simulink library "dspsolvers"  (Simulink 8.0)
settings: Solver=ode45  SolverMode=SingleTasking  StartTime=0.0  StopTime=10.0  RelTol=1e-3
values from neighbouring files (symbols this model uses):
  D = D + B    [rebuffer_delay.m]
libraries: dspsigattribs x12, dspsolvers x6, dspfactors x3, dspmtrx3 x3, dspinverses x1
settings Model: Creator=dlinebar  LastModifiedBy=amoyer  CovMetricSettings=d  ExtModeAutoUpdateStatusClock=off

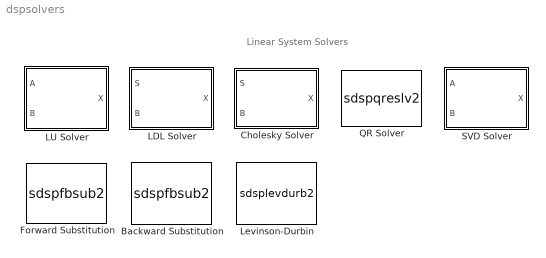
== system dspsolvers ==
  note: Linear System Solvers
  Backward Substitution : S-Function  DialogController=SPCUnifiedFixptDlgDDG.FBSubst  DialogControllerArgs=DataTag0  FunctionName=sdspfbsub2  Parameters=Unit,RealDiag,1,outputMin,outputMax,dtInfo.prodOutputMode,dtInfo.prodOutputWordLength,dtInfo.prodOutputFracLength,dtInfo.accumMode,dtInfo.accumWordLength,dtInfo.accumFracLength,dtInfo.outputMode,dtInfo.outputWordLength,dtInfo.outputFracLength,dtInfo.roundingMode,dtInfo.overflowMode  EnableBusSupport=off  mask(Backward Substitution){Unit=off, RealDiag=off, outputMode=Same as first input, outputWordLength=16, outputFracLength=15, outputDataTypeStr=Inherit: Same as first input, outputLastDataTypeStr=Inherit: Same as first input, outputMin=[], outputMax=[], accumMode=Inherit via internal rule, accumWordLength=32, accumFracLength=30, accumDataTypeStr=Inherit: Inherit via internal rule, accumLastDataTypeStr=Inherit: Inherit via internal rule, prodOutputMode=Inherit via internal rule, prodOutputWordLength=32, prodOutputFracLength=30, prodOutputDataTypeStr=Inherit: Inherit via internal rule, prodOutputLastDataTypeStr=Inherit: Inherit via internal rule, roundingMode=Floor, overflowMode=off, LockScale=off}
      mask prompts: Unit "Input U is unit-upper triangular"; RealDiag "Diagonal of complex input U is real"; outputMode "Fixed-point output attributes:"; outputWordLength "Output word length:"; outputFracLength "Output fraction length:"; outputDataTypeStr "Output data type:"; outputLastDataTypeStr "Last output data type:"; outputMin "Output minimum:"; outputMax "Output maximum:"; accumMode "Fixed-point accumulator attributes:"; accumWordLength "Accumulator word length:"; accumFracLength "Accumulator fraction length:"; accumDataTypeStr "Accumulator data type:"; accumLastDataTypeStr "Last accumulator data type:"; prodOutputMode "Fixed-point product output attributes:"; prodOutputWordLength "Product output word length:"; prodOutputFracLength "Product output fraction length:"; prodOutputDataTypeStr "Product output data type:"; prodOutputLastDataTypeStr "Last product output data type:"; roundingMode "Round integer calculations toward:"; overflowMode "Saturate on integer overflow:"; LockScale "Lock scaling"
      mask help: dsp:dspsolvers:BackwardSubstitution_MD
      mask init:
      | blkh   = gcbh;
      | dtRows = dspblkGetFBSubstDTRowInfo();
      | dtInfo = dspGetUDTFixptDataTypeInfo(blkh, dtRows, true);
      mask Help: eval('blocksethelp');
      mask TypeOptions outputMode: Same as first input | Binary point scaling | Slope and bias scaling
      mask TypeOptions accumMode: Inherit via internal rule | Same as product output | Same as first input | Binary point scaling | Slope and bias scaling
      mask TypeOptions prodOutputMode: Inherit via internal rule | Same as first input | Binary point scaling | Slope and bias scaling
      mask TypeOptions roundingMode: Ceiling | Convergent | Floor | Nearest | Round | Simplest | Zero
      mask Display:
      | x=[ 0.45 0.45 0.18 0.45 NaN 0.495 0.585 0.585 0.495 0.495 NaN 0.63 0.675 NaN 0.63 0.675 NaN 0.72 0.81 0.81 0.72 0.72 ];
      | y=[ 0.1 0.7 0.7 0.1 NaN 0.1 0.1 0.7 0.7 0.1 NaN 0.35 0.35 NaN 0.45 0.45 NaN 0.1 0.1 0.7 0.7 0.1 ];
      | plot(x,y); text(.4,0.9,'U X = B');
      | port_label('input',1,'U');
      | port_label('input',2,'B');
      | port_label('output',1,'X');
  Cholesky Solver : Subsystem  mask(Cholesky Solver){errmode=Warning}
      mask prompts: errmode "dsp:dspsolvers:NonpositiveDefiniteInput_MP"
      mask help: dsp:dspsolvers:CholeskySolver_MD
      mask init:
      | x=[ 0.135 0.475 .475 0.135 0.135 NaN .135 .475 NaN 0.55 0.64 0.64 0.55  0.55 NaN 0.685 0.73 NaN 0.685 0.73 NaN 0.775 0.865 0.865 0.775 0.775 ];
      | y=[ 0.2 0.2 0.7 0.7 .2 NaN .7 .2 NaN 0.2 0.2 0.7 0.7 0.2 NaN 0.4 0.4 NaN 0.45 0.45 NaN 0.2 0.2 0.7 0.7 0.2 ];
      | set_param([gcb '/Cholesky Factorization'],'MaskTunableValues', {'off'});
      | set_param([gcb '/Cholesky Factorization'],'errmode',get_param(gcb,'errmode'));
      mask Help: eval('blocksethelp');
      mask TypeOptions errmode: dsp:dspsolvers:Ignore_CB | dsp:dspsolvers:Warning_CB | dsp:dspsolvers:Error_CB
      mask Display:
      | plot(x,y+0.05);
      | text(0.17,0.9,'SX=B (Chol)');
      | text(0.12,0.15,'[m x m]');
  Forward Substitution : S-Function  DialogController=SPCUnifiedFixptDlgDDG.FBSubst  DialogControllerArgs=DataTag1  FunctionName=sdspfbsub2  Parameters=Unit,RealDiag,0,outputMin,outputMax,dtInfo.prodOutputMode,dtInfo.prodOutputWordLength,dtInfo.prodOutputFracLength,dtInfo.accumMode,dtInfo.accumWordLength,dtInfo.accumFracLength,dtInfo.outputMode,dtInfo.outputWordLength,dtInfo.outputFracLength,dtInfo.roundingMode,dtInfo.overflowMode  EnableBusSupport=off  mask(Forward Substitution){Unit=off, RealDiag=off, outputMode=Same as first input, outputWordLength=16, outputFracLength=15, outputDataTypeStr=Inherit: Same as first input, outputLastDataTypeStr=Inherit: Same as first input, outputMin=[], outputMax=[], accumMode=Inherit via internal rule, accumWordLength=32, accumFracLength=30, accumDataTypeStr=Inherit: Inherit via internal rule, accumLastDataTypeStr=Inherit: Inherit via internal rule, prodOutputMode=Inherit via internal rule, prodOutputWordLength=32, prodOutputFracLength=30, prodOutputDataTypeStr=Inherit: Inherit via internal rule, prodOutputLastDataTypeStr=Inherit: Inherit via internal rule, roundingMode=Floor, overflowMode=off, LockScale=off}
      mask prompts: Unit "Input L is unit-lower triangular"; RealDiag "Diagonal of complex input L is real"; outputMode "Fixed-point output attributes:"; outputWordLength "Output word length:"; outputFracLength "Output fraction length:"; outputDataTypeStr "Output data type:"; outputLastDataTypeStr "Last output data type:"; outputMin "Output minimum:"; outputMax "Output maximum:"; accumMode "Fixed-point accumulator attributes:"; accumWordLength "Accumulator word length:"; accumFracLength "Accumulator fraction length:"; accumDataTypeStr "Accumulator data type:"; accumLastDataTypeStr "Last accumulator data type:"; prodOutputMode "Fixed-point product output attributes:"; prodOutputWordLength "Product output word length:"; prodOutputFracLength "Product output fraction length:"; prodOutputDataTypeStr "Product output data type:"; prodOutputLastDataTypeStr "Last product output data type:"; roundingMode "Round integer calculations toward:"; overflowMode "Saturate on integer overflow"; LockScale "Lock scaling"
      mask help: dsp:dspsolvers:ForwardSubstitution_MD
      mask init:
      | blkh   = gcbh;
      | dtRows = dspblkGetFBSubstDTRowInfo();
      | dtInfo = dspGetUDTFixptDataTypeInfo(blkh, dtRows, true);
      mask Help: eval('blocksethelp');
      mask TypeOptions outputMode: Same as first input | Binary point scaling | Slope and bias scaling
      mask TypeOptions accumMode: Inherit via internal rule | Same as product output | Same as first input | Binary point scaling | Slope and bias scaling
      mask TypeOptions prodOutputMode: Inherit via internal rule | Same as first input | Binary point scaling | Slope and bias scaling
      mask TypeOptions roundingMode: Ceiling | Convergent | Floor | Nearest | Round | Simplest | Zero
      mask Display:
      | x=[ 0.18 0.45 0.18 0.18 NaN 0.495 0.585 0.585 0.495 0.495 NaN 0.63 0.675 NaN 0.63 0.675 NaN 0.72 0.81 0.81 0.72 0.72 ];
      | y=[ 0.1 0.1 0.7 0.1 NaN 0.1 0.1 0.7 0.7 0.1 NaN 0.35 0.35 NaN 0.45 0.45 NaN 0.1 0.1 0.7 0.7 0.1 ];
      | plot(x,y); text(.4,0.9,'L X = B');
      | port_label('input',1,'L');
      | port_label('input',2,'B');
      | port_label('output',1,'X');
  LDL Solver : Subsystem  mask(LDL Solver){errmode=Warning}
      mask prompts: errmode "dsp:dspsolvers:NonpositiveDefiniteInput_MP"
      mask help: dsp:dspsolvers:LDLSolver_MD
      mask init:
      | Bcols=1;
      | x=[ 0.135 0.475 .475 0.135 0.135 NaN .135 .475 NaN 0.55 0.64 0.64 0.55 0.55 NaN 0.685 0.73 NaN 0.685 0.73 NaN 0.775 0.865 0.865 0.775 0.775 ];
      | y=[ 0.2 0.2 0.7 0.7 0.2 NaN .7 .2 NaN 0.2 0.2 0.7 0.7 0.2 NaN 0.4 0.4 NaN 0.45 0.45 NaN 0.2 0.2 0.7 0.7 0.2 ];
      | %
      | set_param([gcb '/LDL Factorization'],'errmode',get_param(gcb,'errmode'));
      mask Help: eval('blocksethelp');
      mask TypeOptions errmode: dsp:dspsolvers:Ignore_CB | dsp:dspsolvers:Warning_CB | dsp:dspsolvers:Error_CB
      mask Display:
      | plot(x,y+0.05);
      | text(0.17,0.9,'SX=B (LDL'')');
      | text(0.12,0.15,'[m x m]');
  LU Solver : Subsystem  mask(LU Solver){}
      mask help: dsp:dspsolvers:LUSolver_MD
      mask init:
      | x=[ 0.135 .475 0.475 0.135 .135 NaN 0.55 0.64 0.64 0.55 0.55 NaN 0.685 0.73 NaN 0.685 0.73 NaN 0.775 0.865 0.865 0.775 0.775 ];
      | y=[ 0.2 0.2 0.7 0.7 0.2 NaN 0.2 0.2 0.7 0.7 0.2 NaN 0.4 0.4 NaN 0.45 0.45 NaN 0.2 0.2 0.7 0.7 0.2 ];
      mask Help: eval('blocksethelp');
      mask Display:
      | plot(x,y+0.05);
      | 
      | text(0.25,0.9,'AX=B (LU)');
      | 
      | text(0.12,0.15,'[m x m]');
  Levinson-Durbin : S-Function  DialogController=dspDDGCreate  DialogControllerArgs=DataTag2  FunctionName=sdsplevdurb2  Parameters=coeffOutFcnActive,outP,zeroInpHandling,coeffOutFcn,firstCoeffMin,firstCoeffMax,secondCoeffMin,secondCoeffMax,outputMin,outputMax,dtInfo.firstCoeffMode,dtInfo.firstCoeffWordLength,dtInfo.firstCoeffFracLength,dtInfo.secondCoeffMode,dtInfo.secondCoeffWordLength,dtInfo.secondCoeffFracLength,dtInfo.prodOutputMode,dtInfo.prodOutputWordLength,dtInfo.prodOutputFracLength,dtInfo.accumMode,dtInfo.accumWordLength,dtInfo.accumFracLength,dtInfo.outputMode,dtInfo.outputWordLength,dtInfo.outputFracLength,dtInfo.roundingMode,dtInfo.overflowMode  EnableBusSupport=off  mask(Levinson-Durbin){coeffOutFcn=OBSOLETE, coeffOutFcnActive=K, outP=off, zeroInpHandling=on, additionalParams=off, allowOverrides=off, firstCoeffMode=Binary point scaling, firstCoeffWordLength=16, firstCoeffFracLength=0, firstCoeffDataTypeStr=fixdt(1,16,0), firstCoeffLastDataTypeStr=fixdt(1,16,0), firstCoeffMin=[], firstCoeffMax=[], secondCoeffMode=Binary point scaling, secondCoeffWordLength=16, secondCoeffFracLength=0, secondCoeffDataTypeStr=fixdt(1,16,0), secondCoeffLastDataTypeStr=fixdt(1,16,0), secondCoeffMin=[], secondCoeffMax=[], outputMode=Same as input, outputWordLength=16, outputFracLength=15, outputDataTypeStr=Inherit: Same as input, outputLastDataTypeStr=Inherit: Same as input, outputMin=[], outputMax=[], accumMode=Same as input, accumWordLength=32, accumFracLength=30, accumDataTypeStr=Inherit: Same as input, accumLastDataTypeStr=Inherit: Same as input, prodOutputMode=Same as input, prodOutputWordLength=32, prodOutputFracLength=30, prodOutputDataTypeStr=Inherit: Same as input, prodOutputLastDataTypeStr=Inherit: Same as input, roundingMode=Floor, overflowMode=off, LockScale=off}
      mask prompts: coeffOutFcn "Output(s) obsolete:"; coeffOutFcnActive "Output(s):"; outP "Output prediction error power (P)"; zeroInpHandling "If the value of lag 0 is zero, A=[1 zeros], K=[zeros], P=0"; additionalParams "--------------- Show additional parameters ---------------"; allowOverrides "Allow overrides from DSP Attributes blocksAllow overrides from DSP Attributes blocks"; firstCoeffMode "Fixed-point A attributes:"; firstCoeffWordLength "A word length:"; firstCoeffFracLength "A fraction length:"; firstCoeffDataTypeStr "A data type:"; firstCoeffLastDataTypeStr "Last A data type:"; firstCoeffMin "A minimum:"; firstCoeffMax "A maximum:"; secondCoeffMode "Fixed-point K attributes:"; secondCoeffWordLength "K word length:"; secondCoeffFracLength "K fraction length:"; secondCoeffDataTypeStr "K data type:"; secondCoeffLastDataTypeStr "Last K data type:"; secondCoeffMin "K minimum:"; secondCoeffMax "K maximum:"; outputMode "Fixed-point P attributes:"; outputWordLength "P word length:"; outputFracLength "P fractional length:"; outputDataTypeStr "P data type:"; outputLastDataTypeStr "Last P data type:"; outputMin "P minimum:"; outputMax "P maximum:"; accumMode "Fixed-point accumulator attributes:"; accumWordLength "Accumulator word length:"; accumFracLength "Accumulator fraction length:"; accumDataTypeStr "Accumulator data type:"; accumLastDataTypeStr "Last accumulator data type:"; prodOutputMode "Fixed-point product output attributes:"; prodOutputWordLength "Product output word length:"; prodOutputFracLength "Product output fraction length:"; prodOutputDataTypeStr "Product output data type:"; prodOutputLastDataTypeStr "Last product output data type:"; roundingMode "Round integer calculations towards:"; overflowMode "Saturate on integer overflow"; LockScale "Lock scaling"
      mask help: dsp:dspsolvers:LevinsonDurbin_MD
      mask init:
      | blkh   = gcbh;
      | dspblklevdurb2();
      | dtRows = dspblkGetLevDurbDTRowInfo();
      | dtInfo = dspGetUDTFixptDataTypeInfo(blkh, dtRows, true);
      mask Help: eval('blocksethelp');
      mask TypeOptions coeffOutFcn: A and K | A | K | OBSOLETE
      mask TypeOptions coeffOutFcnActive: A and K | A | K
      mask TypeOptions firstCoeffMode: Binary point scaling | Slope and bias scaling | User-defined
      mask TypeOptions secondCoeffMode: Binary point scaling | Slope and bias scaling | User-defined
      mask TypeOptions outputMode: Same as input | Binary point scaling | Slope and bias scaling | User-defined
      mask TypeOptions accumMode: Same as product output | Same as input | Binary point scaling | Slope and bias scaling | User-defined
      mask TypeOptions prodOutputMode: Same as input | Binary point scaling | Slope and bias scaling | User-defined
      mask TypeOptions roundingMode: Ceiling | Convergent | Floor | Nearest | Round | Simplest | Zero
      mask Display:
      | text(0.2,0.6,'Levinson-');
      | text(0.3,0.4,'Durbin');
      | 
      | s    = [];
      | s.o1 = 1; s.o1s = '';
      | s.o2 = 1; s.o2s = '';
      | s.o3 = 1; s.o3s = '';
      | 
      | switch coeffOutFcnActive
      | case 1 % CASE: A and K
      |     if (outP == 1) % 3 outputs (A,K,P)
      |         s.o1 = 1; s.o1s = 'A';
      |         s.o2 = 2; s.o2s = 'K';
      |         s.o3 = 3; s.o3s = 'P';
      |     else % 2 outputs (A,K)
      |         s.o2 = 1; s.o2s = 'A';
      |         s.o3 = 2; s.o3s = 'K';
      |     end
      | case 2 % CASE: A
      |     if (outP == 1) % 2 outputs (A,P)
      |         s.o2 = 1; s.o2s = 'A';
      |         s.o3 = 2; s.o3s = 'P';
      |     else % 1 output (A)
      |         s.o3 = 1; s.o3s = 'A';
      |     end
      | otherwise % CASE: K
      |     if (outP == 1) % 2 outputs (K,P)
      |         s.o2 = 1; s.o2s = 'K';
      |         s.o3 = 2; s.o3s = 'P';
      |     else % 1 output (K)
      |         s.o3 = 1; s.o3s = 'K';
      |     end
      | end
      | 
      | port_label('output',s.o1,s.o1s);
      | port_label('output',s.o2,s.o2s);
      | port_label('output',s.o3,s.o3s);
  QR Solver : S-Function  FunctionName=sdspqreslv2  EnableBusSupport=off  mask(QR Solver){}
      mask help: dsp:dspsolvers:QRSolver_MD
      mask init:
      | x=[ 0.2 0.475 .475 0.2 0.2 NaN 0.55 0.64 0.64 0.55 0.55 NaN 0.685 0.73 NaN 0.685 0.73 NaN 0.775 0.865 0.865 0.775 0.775 ];
      | y=[ 0.2 0.2 0.7 0.7 0.2 NaN 0.35 0.35 0.7 0.7 0.35 NaN 0.4 0.4 NaN 0.45 0.45 NaN 0.2 0.2 0.7 0.7 0.2 ];
      mask Help: eval('blocksethelp');
      mask Display:
      | plot(x,y+0.05);
      | text(0.23,0.9,'AX=B (QR)');
      | text(0.17,0.15,'[m x n]');
      | port_label('input',1,'A');
      | port_label('input',2,'B');
      | port_label('output',1,'X');
  SVD Solver : Subsystem  mask(SVD Solver){wanterr=off}
      mask prompts: wanterr "dsp:dspsolvers:ShowErrorStatusPortE_MP"
      mask help: dsp:dspsolvers:SVDSolver_MD
      mask init:
      | x=[ 0.2 0.475 .475 0.2 0.2 NaN 0.55 0.64 0.64 0.55 0.55 NaN 0.685 0.73 NaN 0.685 0.73 NaN 0.775 0.865 0.865 0.775 0.775 ];
      | y=[ 0.2 0.2 0.7 0.7 0.2 NaN 0.35 0.35 0.7 0.7 0.35 NaN 0.4 0.4 NaN 0.45 0.45 NaN 0.2 0.2 0.7 0.7 0.2 ];
      | 
      | blk = gcb;
      | 
      | % The error port output block
      | errBlk      = [blk '/E'];
      | portList = get_param(blk,'Ports');
      | portPresent = (portList(2) == 2);
      | 
      | if (wanterr)
      |     % Turn the error port on in the pinv block
      |     set_param([blk , '/Pseudoinverse'], 'wanterr', 'on');
      |     
      |     if (~portPresent)
      |         % Add the outport and connect it
      |         add_block('built-in/Outport', errBlk, ...,
      |             'Position', [355   115   375   135 ]);
      |         add_line(blk, 'Pseudoinverse/2', 'E/1');
      |     end
      | else
      |     if (portPresent)
      |         % Delete the error outport and the connection to it
      |         delete_line(blk, 'Pseudoinverse/2', 'E/1');
      |         delete_block(errBlk);
      |     end
      |     % Turn off the error port on the pinv block
      |     set_param([blk , '/Pseudoinverse'], 'wanterr', 'off');
      | end
      mask Help: eval('blocksethelp');
      mask Display:
      | plot(x,y+0.05);
      | 
      | text(0.2,0.9,'AX=B (SVD)');
      | 
      | text(0.17,0.15,'[m x n]');

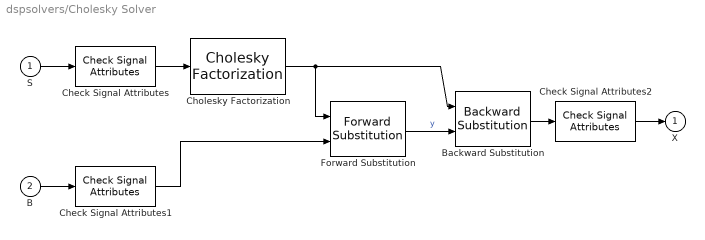
== system dspsolvers/Cholesky Solver ==
  S : Inport
  B : Inport  Port=2
  Backward Substitution : dspsolvers/Backward Substitution  Unit=off  RealDiag=off  outputMin=[]  outputMax=[]  accumDataTypeStr=Inherit: Same as product output  accumLastDataTypeStr=Inherit: Same as product output  roundingMode=Floor  overflowMode=off
  Check Signal Attributes : dspsigattribs/Check Signal Attributes  SystemSampleTime=-1  SigAttribCheckMethod=Does not match attributes exactly  Complexity=Ignore  Frame=Ignore  DimsCheckMethod=Ignore  Dimensions=1-D  DatatypeCheckMethod=Is...  DatatypeGeneral=Floating-point  DtypeFloatSpecific=Any floating-point  DtypeFixedSpecific=Any fixed-point  DtypeIntSpecific=Any integer  SampleMode=Ignore
  Check Signal Attributes1 : dspsigattribs/Check Signal Attributes  SystemSampleTime=-1  SigAttribCheckMethod=Does not match attributes exactly  Complexity=Ignore  Frame=Ignore  DimsCheckMethod=Ignore  Dimensions=1-D  DatatypeCheckMethod=Is...  DatatypeGeneral=Floating-point  DtypeFloatSpecific=Any floating-point  DtypeFixedSpecific=Any fixed-point  DtypeIntSpecific=Any integer  SampleMode=Ignore
  Check Signal Attributes2 : dspsigattribs/Check Signal Attributes  SystemSampleTime=-1  SigAttribCheckMethod=Does not match attributes exactly  Complexity=Ignore  Frame=Ignore  DimsCheckMethod=Ignore  Dimensions=1-D  DatatypeCheckMethod=Is...  DatatypeGeneral=Floating-point  DtypeFloatSpecific=Any floating-point  DtypeFixedSpecific=Any fixed-point  DtypeIntSpecific=Any integer  SampleMode=Ignore
  Cholesky Factorization : dspfactors/Cholesky Factorization  errmode=Warning
  Forward Substitution : dspsolvers/Forward Substitution  Unit=off  RealDiag=off  outputMin=[]  outputMax=[]  accumDataTypeStr=Inherit: Same as product output  accumLastDataTypeStr=Inherit: Same as product output  roundingMode=Floor  overflowMode=off
  X : Outport  InitialOutput=0
  wires:
  S/1 -> Check Signal Attributes/1
  Forward Substitution/1 -> Backward Substitution/2  "y"
  Backward Substitution/1 -> Check Signal Attributes2/1
  Cholesky Factorization/1 -> Forward Substitution/1, Backward Substitution/1
  Check Signal Attributes/1 -> Cholesky Factorization/1
  B/1 -> Check Signal Attributes1/1
  Check Signal Attributes1/1 -> Forward Substitution/2
  Check Signal Attributes2/1 -> X/1

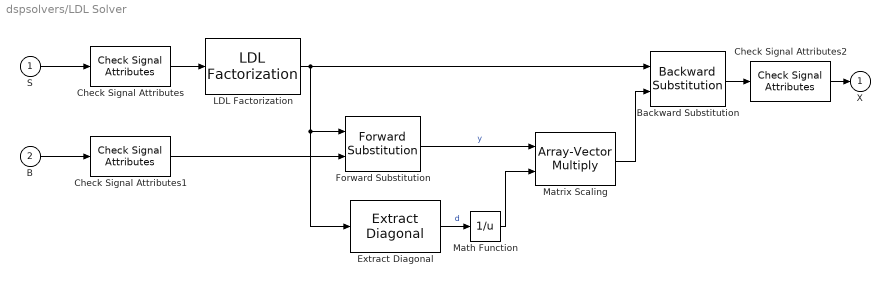
== system dspsolvers/LDL Solver ==
  S : Inport
  B : Inport  Port=2
  Backward Substitution : dspsolvers/Backward Substitution  Unit=on  RealDiag=on  outputMin=[]  outputMax=[]  accumDataTypeStr=Inherit: Same as product output  accumLastDataTypeStr=Inherit: Same as product output  roundingMode=Floor  overflowMode=off
  Check Signal Attributes : dspsigattribs/Check Signal Attributes  SystemSampleTime=-1  SigAttribCheckMethod=Does not match attributes exactly  Complexity=Ignore  Frame=Ignore  DimsCheckMethod=Ignore  Dimensions=1-D  DatatypeCheckMethod=Is...  DatatypeGeneral=Floating-point  DtypeFloatSpecific=Any floating-point  DtypeFixedSpecific=Any fixed-point  DtypeIntSpecific=Any integer  SampleMode=Ignore
  Check Signal Attributes1 : dspsigattribs/Check Signal Attributes  SystemSampleTime=-1  SigAttribCheckMethod=Does not match attributes exactly  Complexity=Ignore  Frame=Ignore  DimsCheckMethod=Ignore  Dimensions=1-D  DatatypeCheckMethod=Is...  DatatypeGeneral=Floating-point  DtypeFloatSpecific=Any floating-point  DtypeFixedSpecific=Any fixed-point  DtypeIntSpecific=Any integer  SampleMode=Ignore
  Check Signal Attributes2 : dspsigattribs/Check Signal Attributes  SystemSampleTime=-1  SigAttribCheckMethod=Does not match attributes exactly  Complexity=Ignore  Frame=Ignore  DimsCheckMethod=Ignore  Dimensions=1-D  DatatypeCheckMethod=Is...  DatatypeGeneral=Floating-point  DtypeFloatSpecific=Any floating-point  DtypeFixedSpecific=Any fixed-point  DtypeIntSpecific=Any integer  SampleMode=Ignore
  Extract Diagonal : dspmtrx3/Extract Diagonal
  Forward Substitution : dspsolvers/Forward Substitution  Unit=on  RealDiag=on  outputMin=[]  outputMax=[]  accumDataTypeStr=Inherit: Same as product output  accumLastDataTypeStr=Inherit: Same as product output  roundingMode=Floor  overflowMode=off
  LDL Factorization : dspfactors/LDL Factorization  errmode=Warning  outputMin=[]  outputMax=[]  roundingMode=Floor  overflowMode=off
  Math Function : Math  Operator=reciprocal  SaturateOnIntegerOverflow=on
  Matrix Scaling : dspmtrx3/Array-Vector Multiply  mode=Mute  saveAsFlag=0  Dimension=1  V_Source=Input port  V_VectFromMask=[0.5 0.25]  firstCoeffSignedness=Auto  firstCoeffDataTypeStr=Inherit: Same word length as input  firstCoeffLastDataTypeStr=Inherit: Same word length as input  firstCoeffMin=[]  firstCoeffMax=[]  outputSignedness=Auto  outputDataTypeStr=Inherit: Same as product output  outputLastDataTypeStr=Inherit: Same as product output  outputMin=[]  outputMax=[]  accumSignedness=Auto  prodOutputSignedness=Auto  roundingMode=Floor  overflowMode=off
  X : Outport  InitialOutput=0
  wires:
  Backward Substitution/1 -> Check Signal Attributes2/1
  LDL Factorization/1 -> Backward Substitution/1, Forward Substitution/1, Extract Diagonal/1
  B/1 -> Check Signal Attributes1/1
  S/1 -> Check Signal Attributes/1
  Forward Substitution/1 -> Matrix Scaling/1  "y"
  Matrix Scaling/1 -> Backward Substitution/2
  Extract Diagonal/1 -> Math Function/1  "d"
  Math Function/1 -> Matrix Scaling/2
  Check Signal Attributes/1 -> LDL Factorization/1
  Check Signal Attributes1/1 -> Forward Substitution/2
  Check Signal Attributes2/1 -> X/1

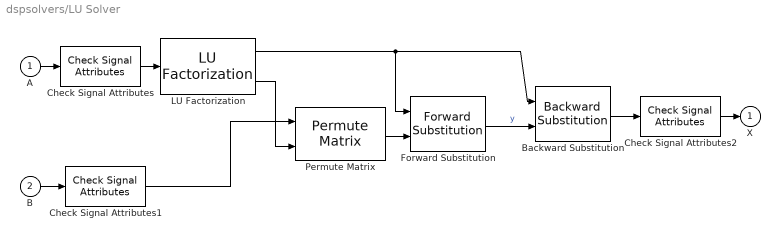
== system dspsolvers/LU Solver ==
  A : Inport
  B : Inport  Port=2
  Backward Substitution : dspsolvers/Backward Substitution  Unit=off  RealDiag=off  outputMin=[]  outputMax=[]  accumDataTypeStr=Inherit: Same as product output  accumLastDataTypeStr=Inherit: Same as product output  roundingMode=Floor  overflowMode=off
  Check Signal Attributes : dspsigattribs/Check Signal Attributes  SystemSampleTime=-1  SigAttribCheckMethod=Does not match attributes exactly  Complexity=Ignore  Frame=Ignore  DimsCheckMethod=Ignore  Dimensions=1-D  DatatypeCheckMethod=Is...  DatatypeGeneral=Floating-point  DtypeFloatSpecific=Any floating-point  DtypeFixedSpecific=Any fixed-point  DtypeIntSpecific=Any integer  SampleMode=Ignore
  Check Signal Attributes1 : dspsigattribs/Check Signal Attributes  SystemSampleTime=-1  SigAttribCheckMethod=Does not match attributes exactly  Complexity=Ignore  Frame=Ignore  DimsCheckMethod=Ignore  Dimensions=1-D  DatatypeCheckMethod=Is...  DatatypeGeneral=Floating-point  DtypeFloatSpecific=Any floating-point  DtypeFixedSpecific=Any fixed-point  DtypeIntSpecific=Any integer  SampleMode=Ignore
  Check Signal Attributes2 : dspsigattribs/Check Signal Attributes  SystemSampleTime=-1  SigAttribCheckMethod=Does not match attributes exactly  Complexity=Ignore  Frame=Ignore  DimsCheckMethod=Ignore  Dimensions=1-D  DatatypeCheckMethod=Is...  DatatypeGeneral=Floating-point  DtypeFloatSpecific=Any floating-point  DtypeFixedSpecific=Any fixed-point  DtypeIntSpecific=Any integer  SampleMode=Ignore
  Forward Substitution : dspsolvers/Forward Substitution  Unit=on  RealDiag=on  outputMin=[]  outputMax=[]  accumDataTypeStr=Inherit: Same as product output  accumLastDataTypeStr=Inherit: Same as product output  roundingMode=Floor  overflowMode=off
  LU Factorization : dspfactors/LU Factorization  singular=off  outputMin=[]  outputMax=[]  roundingMode=Floor  overflowMode=off
  Permute Matrix : dspmtrx3/Permute Matrix  mode=Rows  ZeroOneIdxMode=One-based  errmode=Clip index  checkDims=on
  X : Outport  InitialOutput=0
  wires:
  A/1 -> Check Signal Attributes/1
  Permute Matrix/1 -> Forward Substitution/2
  Backward Substitution/1 -> Check Signal Attributes2/1
  Forward Substitution/1 -> Backward Substitution/2  "y"
  B/1 -> Check Signal Attributes1/1
  LU Factorization/2 -> Permute Matrix/2
  LU Factorization/1 -> Forward Substitution/1, Backward Substitution/1
  Check Signal Attributes/1 -> LU Factorization/1
  Check Signal Attributes1/1 -> Permute Matrix/1
  Check Signal Attributes2/1 -> X/1

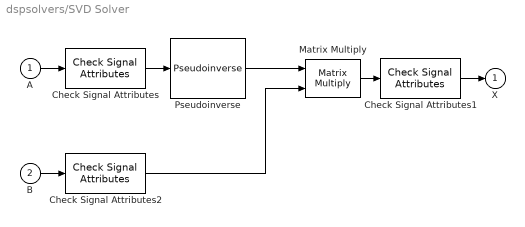
== system dspsolvers/SVD Solver ==
  A : Inport
  B : Inport  Port=2
  Check Signal Attributes : dspsigattribs/Check Signal Attributes  SystemSampleTime=-1  SigAttribCheckMethod=Does not match attributes exactly  Complexity=Ignore  Frame=Ignore  DimsCheckMethod=Ignore  Dimensions=1-D  DatatypeCheckMethod=Is...  DatatypeGeneral=Floating-point  DtypeFloatSpecific=Any floating-point  DtypeFixedSpecific=Any fixed-point  DtypeIntSpecific=Any integer  SampleMode=Ignore
  Check Signal Attributes1 : dspsigattribs/Check Signal Attributes  SystemSampleTime=-1  SigAttribCheckMethod=Does not match attributes exactly  Complexity=Ignore  Frame=Ignore  DimsCheckMethod=Ignore  Dimensions=1-D  DatatypeCheckMethod=Is...  DatatypeGeneral=Floating-point  DtypeFloatSpecific=Any floating-point  DtypeFixedSpecific=Any fixed-point  DtypeIntSpecific=Any integer  SampleMode=Ignore
  Check Signal Attributes2 : dspsigattribs/Check Signal Attributes  SystemSampleTime=-1  SigAttribCheckMethod=Does not match attributes exactly  Complexity=Ignore  Frame=Ignore  DimsCheckMethod=Ignore  Dimensions=1-D  DatatypeCheckMethod=Is...  DatatypeGeneral=Floating-point  DtypeFloatSpecific=Any floating-point  DtypeFixedSpecific=Any fixed-point  DtypeIntSpecific=Any integer  SampleMode=Ignore
  Matrix Multiply : Product  Multiplication=Matrix(*)
  Pseudoinverse : dspinverses/Pseudoinverse  wanterr=off
  X : Outport  InitialOutput=0
  wires:
  A/1 -> Check Signal Attributes/1
  Pseudoinverse/1 -> Matrix Multiply/1
  Matrix Multiply/1 -> Check Signal Attributes1/1
  B/1 -> Check Signal Attributes2/1
  Check Signal Attributes/1 -> Pseudoinverse/1
  Check Signal Attributes1/1 -> X/1
  Check Signal Attributes2/1 -> Matrix Multiply/2
